simulink subsystem "Bus_phasor"  (R2020a)
settings: Solver=VariableStepAuto  StartTime=0.0  StopTime=10.0  RelTol=1e-3
libraries: powerlib_meascontrol x1, powerlib x1
settings Model: Creator=anton  LastModifiedBy=anton
settings DebuggingCC: SFMachineParentedDataDiag=error

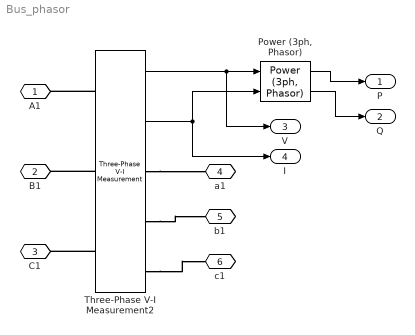
== system Bus_phasor ==
  "Power (3ph, Phasor)" : powerlib_meascontrol/Measurements/Power (3ph, Phasor)
      settings: SourceProductBaseCode=PS
  Three-Phase V-I Measurement2 : powerlib/Measurements/Three-Phase V-I Measurement  VoltageMeasurement=phase-to-ground  SetLabelV=off  LabelV=Vabc  Vpu=off  VpuLL=off  CurrentMeasurement=yes  SetLabelI=off  LabelI=Iabc  Ipu=off  Pbase=100e6  Vbase=500e3  OutputType=Complex  PhasorSimulation=on  PSBequivalent=0
  A1 : PMIOPort  Side=Left
  B1 : PMIOPort  Port=2  Side=Left
  C1 : PMIOPort  Port=3  Side=Left
  a1 : PMIOPort  Port=4  Side=Right
  b1 : PMIOPort  Port=5  Side=Right
  c1 : PMIOPort  Port=6  Side=Right
  P : Outport
  Q : Outport  Port=2
  V : Outport  Port=3
  I : Outport  Port=4
  wires:
  Three-Phase V-I Measurement2/1 -> V/1, "Power (3ph, Phasor)"/1
  Three-Phase V-I Measurement2/2 -> "Power (3ph, Phasor)"/2, I/1
  "Power (3ph, Phasor)"/1 -> P/1
  "Power (3ph, Phasor)"/2 -> Q/1
  connections:
  Three-Phase V-I Measurement2/LConn3 -- C1/RConn1
  Three-Phase V-I Measurement2/LConn1 -- A1/RConn1
  Three-Phase V-I Measurement2/RConn1 -- a1/RConn1
  Three-Phase V-I Measurement2/RConn3 -- c1/RConn1
  Three-Phase V-I Measurement2/RConn2 -- b1/RConn1
  Three-Phase V-I Measurement2/LConn2 -- B1/RConn1
